simulink model "EX2"  (R2020a)
settings: Solver=ode23  StartTime=0.0  StopTime=10.0  RelTol=1e-3
PostLoadFcn:
  | Fn=[0 0;1 0.8;2 1.6;3 1.6;4 1.6;5 1.6;6 0.8;7 0;8 0;9 0;10 0];
  | le=1;
  | lv=5;
  | R=1;
  | Tin=[1 2;2 2;3 2;4 2;5 2;6 0;7 0;8 0;9 0;10 0];
  | be=2;
  | bv=1;
  | f1=[1;6;11;16;21;26;31;36;41;46;51];
  | muk=1;
  | mus=1.5;
model workspace (MAT data in the model file):
  Fn = [0  0; 1  0.8; 2  1.6; 3  1.6; 4  1.6; 5  1.6; 6  0.8; 7  0; 8  0; 9  0; 10  0]
  R = 1
  Tin = [1  2; 2  2; 3  2; 4  2; 5  2; 6  0; 7  0; 8  0; 9  0; 10  0]
  be = 2
  bv = 1
  f1 = [1; 6; 11; 16; 21; 26; 31; 26; 41; 46; 51]
  le = 1
  lv = 5
  muk = 1
  mus = 1.5
settings Model: DataDictionary=clutch_data.sldd  Creator=aishw  LastModifiedBy=aishw

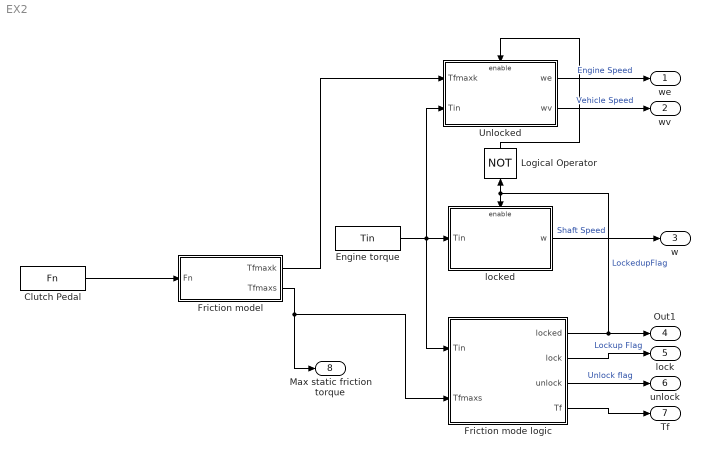
== system EX2 ==
  Clutch Pedal : FromWorkspace  VariableName=Fn  ZeroCross=off
  Engine torque : FromWorkspace  VariableName=Tin  ZeroCross=off
  Friction mode logic : Subsystem
  Friction model : Subsystem
  Logical Operator : Logic  Operator=NOT  IconShape=distinctive  AllPortsSameDT=off  OutDataTypeStr=boolean
  Unlocked : Subsystem
  locked : Subsystem
  we : Outport
  wv : Outport  Port=2
  w : Outport  Port=3
  Out1 : Outport  Port=4
  lock : Outport  Port=5
  unlock : Outport  Port=6
  Tf : Outport  Port=7
  Max static friction torque : Outport  Port=8
  wires:
  Clutch Pedal/1 -> Friction model/1(Fn)
  Unlocked/1(we) -> we/1  "Engine Speed"
  Unlocked/2(wv) -> wv/1  "Vehicle Speed"
  Logical Operator/1 -> Unlocked/Enable
  Engine torque/1 -> Unlocked/2(Tin), Friction mode logic/1(Tin), locked/1(Tin)
  Friction model/2(Tfmaxs) -> Max static friction torque/1, Friction mode logic/2(Tfmaxs)
  locked/1(w) -> w/1  "Shaft Speed"
  Friction mode logic/2(lock) -> lock/1  "Lockup Flag"
  Friction mode logic/4(Tf) -> Tf/1
  Friction mode logic/3(unlock) -> unlock/1  "Unlock flag"
  Friction mode logic/1(locked) -> locked/Enable, Logical Operator/1, Out1/1  "LockedupFlag"
  Friction model/1(Tfmaxk) -> Unlocked/1(Tfmaxk)

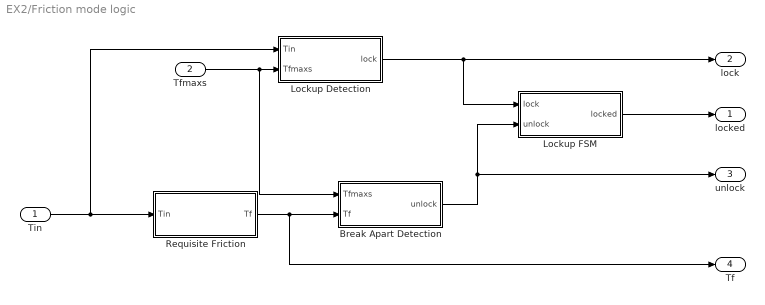
== system EX2/Friction mode logic ==
  Tin : Inport
  Tfmaxs : Inport  Port=2
  Break Apart Detection : Subsystem
  Lockup Detection : Subsystem
  "Lockup FSM " : Subsystem
  Requisite Friction : Subsystem
  locked : Outport
  lock : Outport  Port=2
  unlock : Outport  Port=3
  Tf : Outport  Port=4
  wires:
  "Lockup FSM "/1(locked) -> locked/1
  Break Apart Detection/1(unlock) -> "Lockup FSM "/2(unlock), unlock/1
  Lockup Detection/1(lock) -> "Lockup FSM "/1(lock), lock/1
  Tin/1 -> Lockup Detection/1(Tin), Requisite Friction/1(Tin)
  Requisite Friction/1(Tf) -> Tf/1, Break Apart Detection/2(Tf)
  Tfmaxs/1 -> Break Apart Detection/1(Tfmaxs), Lockup Detection/2(Tfmaxs)

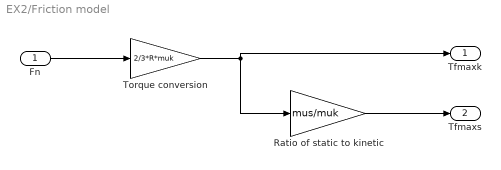
== system EX2/Friction model ==
  Fn : Inport
  Ratio of static to kinetic : Gain  Gain=mus/muk
  Torque conversion : Gain  Gain=2/3*R*muk
  Tfmaxk : Outport
  Tfmaxs : Outport  Port=2
  wires:
  Fn/1 -> Torque conversion/1
  Ratio of static to kinetic/1 -> Tfmaxs/1
  Torque conversion/1 -> Tfmaxk/1, Ratio of static to kinetic/1

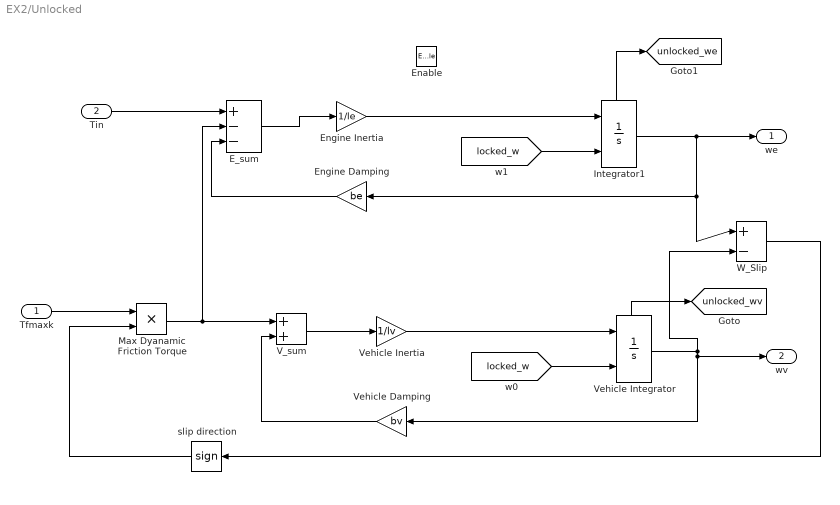
== system EX2/Unlocked ==
  Tfmaxk : Inport
  Tin : Inport  Port=2
  Enable : EnablePort
  E_sum : Sum  Inputs=+--
  Engine Damping : Gain  Gain=be
  Engine Inertia : Gain  Gain=1/le
  Integrator1 : Integrator  InitialConditionSource=external  ShowStatePort=on
  Max Dyanamic Friction Torque : Product
  V_sum : Sum
  Vehicle Damping : Gain  Gain=bv
  Vehicle Inertia : Gain  Gain=1/lv
  Vehicle Integrator : Integrator  InitialConditionSource=external  ShowStatePort=on
  W_Slip : Sum  Inputs=|+-
  slip direction : Signum
  we : Outport
  wv : Outport  Port=2
  tag scope: unlocked_we=global, unlocked_wv=global
  wires:
  Tfmaxk/1 -> Max Dyanamic Friction Torque/1
  slip direction/1 -> Max Dyanamic Friction Torque/2
  Tin/1 -> E_sum/1
  Max Dyanamic Friction Torque/1 -> V_sum/1, E_sum/2
  V_sum/1 -> Vehicle Inertia/1
  E_sum/1 -> Engine Inertia/1
  Engine Damping/1 -> E_sum/3
  Vehicle Damping/1 -> V_sum/2
  Vehicle Inertia/1 -> Vehicle Integrator/1
  [locked_w] -> Vehicle Integrator/2
  Vehicle Integrator/State -> [unlocked_wv]
  Integrator1/State -> [unlocked_we]
  [locked_w] -> Integrator1/2
  Engine Inertia/1 -> Integrator1/1
  Vehicle Integrator/1 -> Vehicle Damping/1, wv/1, W_Slip/2
  Integrator1/1 -> Engine Damping/1, W_Slip/1, we/1
  W_Slip/1 -> slip direction/1

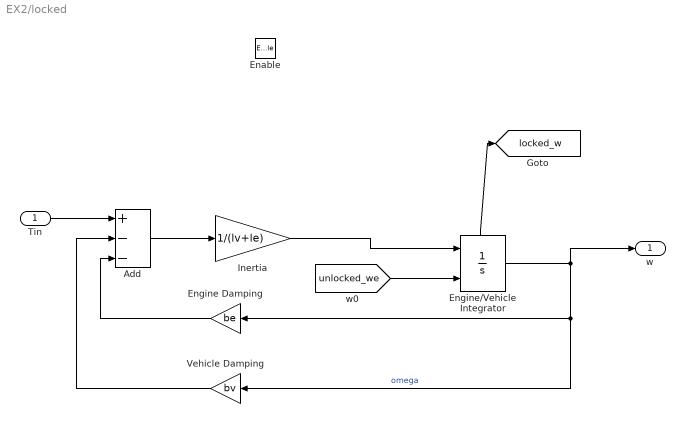
== system EX2/locked ==
  Tin : Inport
  Enable : EnablePort
  Add : Sum  Inputs=+--
  Engine Damping : Gain  Gain=be
  Engine/Vehicle Integrator : Integrator  InitialConditionSource=external  ShowStatePort=on
  Inertia : Gain  Gain=1/(lv+le)
  Vehicle Damping : Gain  Gain=bv
  w : Outport
  tag scope: locked_w=global
  wires:
  Tin/1 -> Add/1
  Add/1 -> Inertia/1
  Engine Damping/1 -> Add/3
  Vehicle Damping/1 -> Add/2
  Inertia/1 -> Engine/Vehicle Integrator/1
  [unlocked_we] -> Engine/Vehicle Integrator/2
  Engine/Vehicle Integrator/1 -> Engine Damping/1, Vehicle Damping/1, w/1  "omega"
  Engine/Vehicle Integrator/State -> [locked_w]

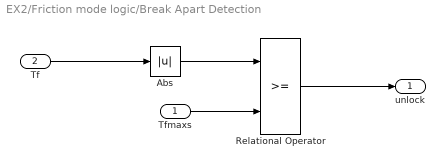
== system EX2/Friction mode logic/Break Apart Detection ==
  Tfmaxs : Inport
  Tf : Inport  Port=2
  Abs : Abs
  Relational Operator : RelationalOperator  OutDataTypeStr=boolean  RndMeth=Simplest
  unlock : Outport
  wires:
  Tf/1 -> Abs/1
  Abs/1 -> Relational Operator/1
  Tfmaxs/1 -> Relational Operator/2
  Relational Operator/1 -> unlock/1

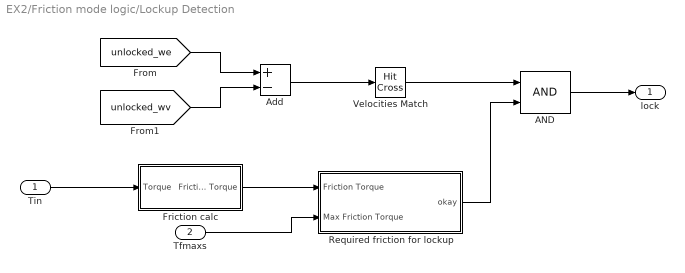
== system EX2/Friction mode logic/Lockup Detection ==
  Tin : Inport
  Tfmaxs : Inport  Port=2
  AND : Logic  IconShape=distinctive  AllPortsSameDT=off  OutDataTypeStr=boolean
  Add : Sum  Inputs=+-
  Friction calc : Subsystem
  Required friction for lockup : Subsystem
  Velocities Match : HitCross
  lock : Outport
  wires:
  Tin/1 -> Friction calc/1(Torque)
  Friction calc/1(Friction Torque) -> Required friction for lockup/1(Friction Torque)
  Tfmaxs/1 -> Required friction for lockup/2(Max Friction Torque)
  [unlocked_we] -> Add/1
  [unlocked_wv] -> Add/2
  Add/1 -> Velocities Match/1
  Velocities Match/1 -> AND/1
  Required friction for lockup/1(okay) -> AND/2
  AND/1 -> lock/1

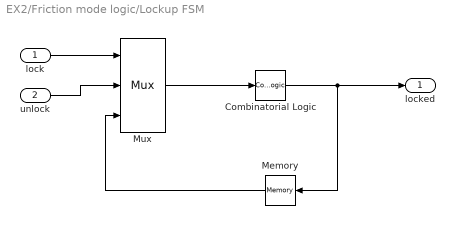
== system EX2/Friction mode logic/Lockup FSM  ==
  lock : Inport
  unlock : Inport  Port=2
  Combinatorial Logic : CombinatorialLogic  TruthTable=[0;1;0;0;1;1;1;0]
  Memory : Memory
  Mux : Mux  Inputs=3
  locked : Outport
  wires:
  Memory/1 -> Mux/3
  unlock/1 -> Mux/2
  lock/1 -> Mux/1
  Mux/1 -> Combinatorial Logic/1
  Combinatorial Logic/1 -> Memory/1, locked/1

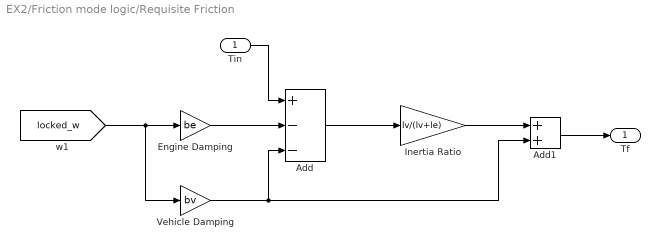
== system EX2/Friction mode logic/Requisite Friction ==
  Tin : Inport
  Add : Sum  Inputs=+--
  Add1 : Sum
  Engine Damping : Gain  Gain=be
  Inertia Ratio : Gain  Gain=lv/(lv+le)
  Vehicle Damping : Gain  Gain=bv
  Tf : Outport
  wires:
  [locked_w] -> Vehicle Damping/1, Engine Damping/1
  Engine Damping/1 -> Add/2
  Tin/1 -> Add/1
  Add/1 -> Inertia Ratio/1
  Inertia Ratio/1 -> Add1/1
  Add1/1 -> Tf/1
  Vehicle Damping/1 -> Add/3, Add1/2

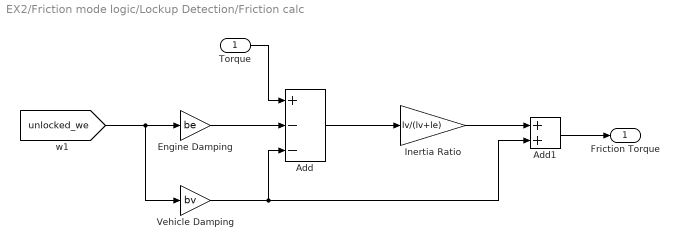
== system EX2/Friction mode logic/Lockup Detection/Friction calc ==
  Torque : Inport
  Add : Sum  Inputs=+--
  Add1 : Sum
  Engine Damping : Gain  Gain=be
  Inertia Ratio : Gain  Gain=lv/(lv+le)
  Vehicle Damping : Gain  Gain=bv
  Friction Torque : Outport
  wires:
  Inertia Ratio/1 -> Add1/1
  [unlocked_we] -> Vehicle Damping/1, Engine Damping/1
  Add/1 -> Inertia Ratio/1
  Engine Damping/1 -> Add/2
  Torque/1 -> Add/1
  Add1/1 -> Friction Torque/1
  Vehicle Damping/1 -> Add/3, Add1/2

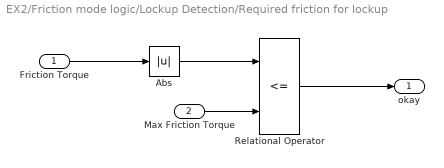
== system EX2/Friction mode logic/Lockup Detection/Required friction for lockup ==
  Friction Torque : Inport
  Max Friction Torque : Inport  Port=2
  Abs : Abs
  Relational Operator : RelationalOperator  Operator=<=  OutDataTypeStr=boolean  RndMeth=Simplest
  okay : Outport
  wires:
  Abs/1 -> Relational Operator/1
  Relational Operator/1 -> okay/1
  Friction Torque/1 -> Abs/1
  Max Friction Torque/1 -> Relational Operator/2
